simulink model "stm32f4_ds3231_configure_demo"  (Simulink 7.3)
settings: Solver=FixedStepDiscrete  SolverMode=SingleTasking  StartTime=0.0  StopTime=10.0  RelTol=1e-3
PreLoadFcn:
  | waijung.modelPreload; % Required for working with Waijung Blockset. Do not remove.
undefined symbols (not defined in the file): HSEOSC, Link, LQFP176, ST, STM32F417IG
libraries: simulink x94, amg_high_precision_rtc x5, stm32f4_io_lib x2, stm32f4_device_config_lib x1
(part 2 of 4)

== system stm32f4_ds3231_configure_demo/Display Date/Time/Display Hour ==
  In1 : Inport
  In2 : Inport  Port=2
  In3 : Inport  Port=3
  Data Type Conversion : DataTypeConversion  OutDataTypeMode=uint8  OutDataType=fixdt(1, 16)  OutScaling=2^0  OutDataTypeStr=uint8
  Logical Operator : Logic  Inputs=3  AllPortsSameDT=off  OutDataTypeMode=boolean  LogicDataType=fixdt(0, 8)  OutDataTypeStr=boolean
  Switch : Switch  Criteria=u2 ~= 0  OutDataType=fixdt(1, 16)  OutScaling=2^0
  Volatile Data Storage Read : S-Function  FunctionName=waijung_vdata_read  Parameters=storagename,varname,sampletime,sampletimestr,blockid,storagetype,storagetypestr  EnableBusSupport=off  mask(waijung_vdata_read){storagename=str_blank2, varname=CharacterLCDSetupVolatileDataStorage7_str_blank2, sampletime=inf, sampletimestr=0.01, blockid=DisplayDateTimeDisplayHourVolatileDataStorageRead, storagetype=string, storagetypestr=uint32_t}
      mask prompts: storagename "Storage Name"; varname "Variable name"; sampletime "Sample time (sec)"; sampletimestr "Compiled sample time (sec) in string"; storagetype "Data type"; storagetypestr "Data type string"
      mask help: This block implements read data from a buffer.
      mask init:
      | waijung_vdata_read_callback('init');
      mask Help: web(fullfile(waijungdocroot,'waijung_vdata_read.htm'))
      mask StyleString: popup(str_hour|str_month|str_year|str_minute|str_second|str_blank2|LCD_Buffer|str_date),edit,edit,edit,edit,edit,edit
      mask CallbackString: waijung_vdata_read_callback('storagename');|waijung_vdata_read_callback('varname');|waijung_vdata_read_callback('sampletime');|waijung_vdata_read_callback('sampletimestr');|waijung_vdata_read_callback('blockid');|waijung_vdata_read_callback('storagetype');|
      mask Display: text(0.05, 0.5, 'Buffer: str_blank2','ver','middle','hor','left');port_label('output',1,'D1(string)')
  Volatile Data Storage Read1 : S-Function  FunctionName=waijung_vdata_read  Parameters=storagename,varname,sampletime,sampletimestr,blockid,storagetype,storagetypestr  EnableBusSupport=off  mask(waijung_vdata_read){storagename=str_hour, varname=CharacterLCDSetupVolatileDataStorage1_str_hour, sampletime=inf, sampletimestr=0.01, blockid=DisplayDateTimeDisplayHourVolatileDataStorageRead1, storagetype=string, storagetypestr=uint32_t}
      mask prompts: storagename "Storage Name"; varname "Variable name"; sampletime "Sample time (sec)"; sampletimestr "Compiled sample time (sec) in string"; storagetype "Data type"; storagetypestr "Data type string"
      mask help: This block implements read data from a buffer.
      mask init:
      | waijung_vdata_read_callback('init');
      mask Help: web(fullfile(waijungdocroot,'waijung_vdata_read.htm'))
      mask StyleString: popup(str_hour|str_month|str_year|str_minute|str_second|str_blank2|LCD_Buffer|str_date),edit,edit,edit,edit,edit,edit
      mask CallbackString: waijung_vdata_read_callback('storagename');|waijung_vdata_read_callback('varname');|waijung_vdata_read_callback('sampletime');|waijung_vdata_read_callback('sampletimestr');|waijung_vdata_read_callback('blockid');|waijung_vdata_read_callback('storagetype');|
      mask Display: text(0.05, 0.5, 'Buffer: str_hour','ver','middle','hor','left');port_label('output',1,'D1(string)')
  Out1 : Outport
  wires:
  In3/1 -> Logical Operator/3
  Switch/1 -> Out1/1
  In2/1 -> Logical Operator/2
  In1/1 -> Logical Operator/1
  Volatile Data Storage Read1/1 -> Switch/3
  Volatile Data Storage Read/1 -> Switch/1
  Logical Operator/1 -> Data Type Conversion/1
  Data Type Conversion/1 -> Switch/2

== system stm32f4_ds3231_configure_demo/Display Date/Time/Display Minute ==
  In1 : Inport
  In2 : Inport  Port=2
  In3 : Inport  Port=3
  Data Type Conversion : DataTypeConversion  OutDataTypeMode=uint8  OutDataType=fixdt(1, 16)  OutScaling=2^0  OutDataTypeStr=uint8
  Logical Operator : Logic  Inputs=3  AllPortsSameDT=off  OutDataTypeMode=boolean  LogicDataType=fixdt(0, 8)  OutDataTypeStr=boolean
  Switch : Switch  Criteria=u2 ~= 0  OutDataType=fixdt(1, 16)  OutScaling=2^0
  Volatile Data Storage Read : S-Function  FunctionName=waijung_vdata_read  Parameters=storagename,varname,sampletime,sampletimestr,blockid,storagetype,storagetypestr  EnableBusSupport=off  mask(waijung_vdata_read){storagename=str_blank2, varname=CharacterLCDSetupVolatileDataStorage7_str_blank2, sampletime=inf, sampletimestr=0.01, blockid=DisplayDateTimeDisplayMinuteVolatileDataStorageRead, storagetype=string, storagetypestr=uint32_t}
      mask prompts: storagename "Storage Name"; varname "Variable name"; sampletime "Sample time (sec)"; sampletimestr "Compiled sample time (sec) in string"; storagetype "Data type"; storagetypestr "Data type string"
      mask help: This block implements read data from a buffer.
      mask init:
      | waijung_vdata_read_callback('init');
      mask Help: web(fullfile(waijungdocroot,'waijung_vdata_read.htm'))
      mask StyleString: popup(str_hour|str_month|str_year|str_minute|str_second|str_blank2|LCD_Buffer|str_date),edit,edit,edit,edit,edit,edit
      mask CallbackString: waijung_vdata_read_callback('storagename');|waijung_vdata_read_callback('varname');|waijung_vdata_read_callback('sampletime');|waijung_vdata_read_callback('sampletimestr');|waijung_vdata_read_callback('blockid');|waijung_vdata_read_callback('storagetype');|
      mask Display: text(0.05, 0.5, 'Buffer: str_blank2','ver','middle','hor','left');port_label('output',1,'D1(string)')
  Volatile Data Storage Read1 : S-Function  FunctionName=waijung_vdata_read  Parameters=storagename,varname,sampletime,sampletimestr,blockid,storagetype,storagetypestr  EnableBusSupport=off  mask(waijung_vdata_read){storagename=str_minute, varname=CharacterLCDSetupVolatileDataStorage4_str_minute, sampletime=inf, sampletimestr=0.01, blockid=DisplayDateTimeDisplayMinuteVolatileDataStorageRead1, storagetype=string, storagetypestr=uint32_t}
      mask prompts: storagename "Storage Name"; varname "Variable name"; sampletime "Sample time (sec)"; sampletimestr "Compiled sample time (sec) in string"; storagetype "Data type"; storagetypestr "Data type string"
      mask help: This block implements read data from a buffer.
      mask init:
      | waijung_vdata_read_callback('init');
      mask Help: web(fullfile(waijungdocroot,'waijung_vdata_read.htm'))
      mask StyleString: popup(str_hour|str_month|str_year|str_minute|str_second|str_blank2|LCD_Buffer|str_date),edit,edit,edit,edit,edit,edit
      mask CallbackString: waijung_vdata_read_callback('storagename');|waijung_vdata_read_callback('varname');|waijung_vdata_read_callback('sampletime');|waijung_vdata_read_callback('sampletimestr');|waijung_vdata_read_callback('blockid');|waijung_vdata_read_callback('storagetype');|
      mask Display: text(0.05, 0.5, 'Buffer: str_minute','ver','middle','hor','left');port_label('output',1,'D1(string)')
  Out1 : Outport
  wires:
  Data Type Conversion/1 -> Switch/2
  Logical Operator/1 -> Data Type Conversion/1
  Volatile Data Storage Read/1 -> Switch/1
  Volatile Data Storage Read1/1 -> Switch/3
  In1/1 -> Logical Operator/1
  In2/1 -> Logical Operator/2
  Switch/1 -> Out1/1
  In3/1 -> Logical Operator/3

== system stm32f4_ds3231_configure_demo/Display Date/Time/Display Month ==
  In1 : Inport
  In2 : Inport  Port=2
  In3 : Inport  Port=3
  Data Type Conversion : DataTypeConversion  OutDataTypeMode=uint8  OutDataType=fixdt(1, 16)  OutScaling=2^0  OutDataTypeStr=uint8
  Logical Operator : Logic  Inputs=3  AllPortsSameDT=off  OutDataTypeMode=boolean  LogicDataType=fixdt(0, 8)  OutDataTypeStr=boolean
  Switch : Switch  Criteria=u2 ~= 0  OutDataType=fixdt(1, 16)  OutScaling=2^0
  Volatile Data Storage Read : S-Function  FunctionName=waijung_vdata_read  Parameters=storagename,varname,sampletime,sampletimestr,blockid,storagetype,storagetypestr  EnableBusSupport=off  mask(waijung_vdata_read){storagename=str_blank2, varname=CharacterLCDSetupVolatileDataStorage7_str_blank2, sampletime=inf, sampletimestr=0.01, blockid=DisplayDateTimeDisplayMonthVolatileDataStorageRead, storagetype=string, storagetypestr=uint32_t}
      mask prompts: storagename "Storage Name"; varname "Variable name"; sampletime "Sample time (sec)"; sampletimestr "Compiled sample time (sec) in string"; storagetype "Data type"; storagetypestr "Data type string"
      mask help: This block implements read data from a buffer.
      mask init:
      | waijung_vdata_read_callback('init');
      mask Help: web(fullfile(waijungdocroot,'waijung_vdata_read.htm'))
      mask StyleString: popup(str_hour|str_month|str_year|str_minute|str_second|str_blank2|LCD_Buffer|str_date),edit,edit,edit,edit,edit,edit
      mask CallbackString: waijung_vdata_read_callback('storagename');|waijung_vdata_read_callback('varname');|waijung_vdata_read_callback('sampletime');|waijung_vdata_read_callback('sampletimestr');|waijung_vdata_read_callback('blockid');|waijung_vdata_read_callback('storagetype');|
      mask Display: text(0.05, 0.5, 'Buffer: str_blank2','ver','middle','hor','left');port_label('output',1,'D1(string)')
  Volatile Data Storage Read1 : S-Function  FunctionName=waijung_vdata_read  Parameters=storagename,varname,sampletime,sampletimestr,blockid,storagetype,storagetypestr  EnableBusSupport=off  mask(waijung_vdata_read){storagename=str_month, varname=CharacterLCDSetupVolatileDataStorage2_str_month, sampletime=inf, sampletimestr=0.01, blockid=DisplayDateTimeDisplayMonthVolatileDataStorageRead1, storagetype=string, storagetypestr=uint32_t}
      mask prompts: storagename "Storage Name"; varname "Variable name"; sampletime "Sample time (sec)"; sampletimestr "Compiled sample time (sec) in string"; storagetype "Data type"; storagetypestr "Data type string"
      mask help: This block implements read data from a buffer.
      mask init:
      | waijung_vdata_read_callback('init');
      mask Help: web(fullfile(waijungdocroot,'waijung_vdata_read.htm'))
      mask StyleString: popup(str_hour|str_month|str_year|str_minute|str_second|str_blank2|LCD_Buffer|str_date),edit,edit,edit,edit,edit,edit
      mask CallbackString: waijung_vdata_read_callback('storagename');|waijung_vdata_read_callback('varname');|waijung_vdata_read_callback('sampletime');|waijung_vdata_read_callback('sampletimestr');|waijung_vdata_read_callback('blockid');|waijung_vdata_read_callback('storagetype');|
      mask Display: text(0.05, 0.5, 'Buffer: str_month','ver','middle','hor','left');port_label('output',1,'D1(string)')
  Out1 : Outport
  wires:
  In3/1 -> Logical Operator/3
  Switch/1 -> Out1/1
  In2/1 -> Logical Operator/2
  In1/1 -> Logical Operator/1
  Volatile Data Storage Read1/1 -> Switch/3
  Volatile Data Storage Read/1 -> Switch/1
  Logical Operator/1 -> Data Type Conversion/1
  Data Type Conversion/1 -> Switch/2

== system stm32f4_ds3231_configure_demo/Display Date/Time/Display Second ==
  In1 : Inport
  In2 : Inport  Port=2
  In3 : Inport  Port=3
  Data Type Conversion : DataTypeConversion  OutDataTypeMode=uint8  OutDataType=fixdt(1, 16)  OutScaling=2^0  OutDataTypeStr=uint8
  Logical Operator : Logic  Inputs=3  AllPortsSameDT=off  OutDataTypeMode=boolean  LogicDataType=fixdt(0, 8)  OutDataTypeStr=boolean
  Switch : Switch  Criteria=u2 ~= 0  OutDataType=fixdt(1, 16)  OutScaling=2^0
  Volatile Data Storage Read : S-Function  FunctionName=waijung_vdata_read  Parameters=storagename,varname,sampletime,sampletimestr,blockid,storagetype,storagetypestr  EnableBusSupport=off  mask(waijung_vdata_read){storagename=str_blank2, varname=CharacterLCDSetupVolatileDataStorage7_str_blank2, sampletime=inf, sampletimestr=0.01, blockid=DisplayDateTimeDisplaySecondVolatileDataStorageRead, storagetype=string, storagetypestr=uint32_t}
      mask prompts: storagename "Storage Name"; varname "Variable name"; sampletime "Sample time (sec)"; sampletimestr "Compiled sample time (sec) in string"; storagetype "Data type"; storagetypestr "Data type string"
      mask help: This block implements read data from a buffer.
      mask init:
      | waijung_vdata_read_callback('init');
      mask Help: web(fullfile(waijungdocroot,'waijung_vdata_read.htm'))
      mask StyleString: popup(str_hour|str_month|str_year|str_minute|str_second|str_blank2|LCD_Buffer|str_date),edit,edit,edit,edit,edit,edit
      mask CallbackString: waijung_vdata_read_callback('storagename');|waijung_vdata_read_callback('varname');|waijung_vdata_read_callback('sampletime');|waijung_vdata_read_callback('sampletimestr');|waijung_vdata_read_callback('blockid');|waijung_vdata_read_callback('storagetype');|
      mask Display: text(0.05, 0.5, 'Buffer: str_blank2','ver','middle','hor','left');port_label('output',1,'D1(string)')
  Volatile Data Storage Read1 : S-Function  FunctionName=waijung_vdata_read  Parameters=storagename,varname,sampletime,sampletimestr,blockid,storagetype,storagetypestr  EnableBusSupport=off  mask(waijung_vdata_read){storagename=str_second, varname=CharacterLCDSetupVolatileDataStorage5_str_second, sampletime=inf, sampletimestr=0.01, blockid=DisplayDateTimeDisplaySecondVolatileDataStorageRead1, storagetype=string, storagetypestr=uint32_t}
      mask prompts: storagename "Storage Name"; varname "Variable name"; sampletime "Sample time (sec)"; sampletimestr "Compiled sample time (sec) in string"; storagetype "Data type"; storagetypestr "Data type string"
      mask help: This block implements read data from a buffer.
      mask init:
      | waijung_vdata_read_callback('init');
      mask Help: web(fullfile(waijungdocroot,'waijung_vdata_read.htm'))
      mask StyleString: popup(str_hour|str_month|str_year|str_minute|str_second|str_blank2|LCD_Buffer|str_date),edit,edit,edit,edit,edit,edit
      mask CallbackString: waijung_vdata_read_callback('storagename');|waijung_vdata_read_callback('varname');|waijung_vdata_read_callback('sampletime');|waijung_vdata_read_callback('sampletimestr');|waijung_vdata_read_callback('blockid');|waijung_vdata_read_callback('storagetype');|
      mask Display: text(0.05, 0.5, 'Buffer: str_second','ver','middle','hor','left');port_label('output',1,'D1(string)')
  Out1 : Outport
  wires:
  In3/1 -> Logical Operator/3
  Switch/1 -> Out1/1
  In2/1 -> Logical Operator/2
  In1/1 -> Logical Operator/1
  Volatile Data Storage Read1/1 -> Switch/3
  Volatile Data Storage Read/1 -> Switch/1
  Logical Operator/1 -> Data Type Conversion/1
  Data Type Conversion/1 -> Switch/2

== system stm32f4_ds3231_configure_demo/Display Date/Time/Display Year ==
  In1 : Inport
  In2 : Inport  Port=2
  In3 : Inport  Port=3
  Data Type Conversion : DataTypeConversion  OutDataTypeMode=uint8  OutDataType=fixdt(1, 16)  OutScaling=2^0  OutDataTypeStr=uint8
  Logical Operator : Logic  Inputs=3  AllPortsSameDT=off  OutDataTypeMode=boolean  LogicDataType=fixdt(0, 8)  OutDataTypeStr=boolean
  Switch : Switch  Criteria=u2 ~= 0  OutDataType=fixdt(1, 16)  OutScaling=2^0
  Volatile Data Storage Read : S-Function  FunctionName=waijung_vdata_read  Parameters=storagename,varname,sampletime,sampletimestr,blockid,storagetype,storagetypestr  EnableBusSupport=off  mask(waijung_vdata_read){storagename=str_blank2, varname=CharacterLCDSetupVolatileDataStorage7_str_blank2, sampletime=inf, sampletimestr=0.01, blockid=DisplayDateTimeDisplayYearVolatileDataStorageRead, storagetype=string, storagetypestr=uint32_t}
      mask prompts: storagename "Storage Name"; varname "Variable name"; sampletime "Sample time (sec)"; sampletimestr "Compiled sample time (sec) in string"; storagetype "Data type"; storagetypestr "Data type string"
      mask help: This block implements read data from a buffer.
      mask init:
      | waijung_vdata_read_callback('init');
      mask Help: web(fullfile(waijungdocroot,'waijung_vdata_read.htm'))
      mask StyleString: popup(str_hour|str_month|str_year|str_minute|str_second|str_blank2|LCD_Buffer|str_date),edit,edit,edit,edit,edit,edit
      mask CallbackString: waijung_vdata_read_callback('storagename');|waijung_vdata_read_callback('varname');|waijung_vdata_read_callback('sampletime');|waijung_vdata_read_callback('sampletimestr');|waijung_vdata_read_callback('blockid');|waijung_vdata_read_callback('storagetype');|
      mask Display: text(0.05, 0.5, 'Buffer: str_blank2','ver','middle','hor','left');port_label('output',1,'D1(string)')
  Volatile Data Storage Read1 : S-Function  FunctionName=waijung_vdata_read  Parameters=storagename,varname,sampletime,sampletimestr,blockid,storagetype,storagetypestr  EnableBusSupport=off  mask(waijung_vdata_read){storagename=str_year, varname=CharacterLCDSetupVolatileDataStorage3_str_year, sampletime=inf, sampletimestr=0.01, blockid=DisplayDateTimeDisplayYearVolatileDataStorageRead1, storagetype=string, storagetypestr=uint32_t}
      mask prompts: storagename "Storage Name"; varname "Variable name"; sampletime "Sample time (sec)"; sampletimestr "Compiled sample time (sec) in string"; storagetype "Data type"; storagetypestr "Data type string"
      mask help: This block implements read data from a buffer.
      mask init:
      | waijung_vdata_read_callback('init');
      mask Help: web(fullfile(waijungdocroot,'waijung_vdata_read.htm'))
      mask StyleString: popup(str_hour|str_month|str_year|str_minute|str_second|str_blank2|LCD_Buffer|str_date),edit,edit,edit,edit,edit,edit
      mask CallbackString: waijung_vdata_read_callback('storagename');|waijung_vdata_read_callback('varname');|waijung_vdata_read_callback('sampletime');|waijung_vdata_read_callback('sampletimestr');|waijung_vdata_read_callback('blockid');|waijung_vdata_read_callback('storagetype');|
      mask Display: text(0.05, 0.5, 'Buffer: str_year','ver','middle','hor','left');port_label('output',1,'D1(string)')
  Out1 : Outport
  wires:
  Data Type Conversion/1 -> Switch/2
  Logical Operator/1 -> Data Type Conversion/1
  Volatile Data Storage Read/1 -> Switch/1
  Volatile Data Storage Read1/1 -> Switch/3
  In1/1 -> Logical Operator/1
  In2/1 -> Logical Operator/2
  Switch/1 -> Out1/1
  In3/1 -> Logical Operator/3

== system stm32f4_ds3231_configure_demo/Display Date/Time/Get Date as String ==
  In1 : Inport
  DS3231 Get Date : Subsystem  mask{blockfunction=date, module=1}
      mask prompts: blockfunction "Function"; module "I2C module"
      mask init:
      | amg_high_precision_rtc_callback('init');
      mask StyleString: popup(temp|time|date),popup(1|2|3)
      mask CallbackString: |amg_high_precision_rtc_callback('module');
      mask Display: text(0.5, 0.5, 'Port: I2C1','ver','middle','hor','center');port_label('input', 1,'SlvAddr');port_label('output', 1,'Status');port_label('output', 2,'Day(1-7)');port_label('output', 3,'Date(1-31)');port_label('output', 4,'Month(1-12)');port_label('output', 5,'Year(0-99)');
  Printf1 : S-Function  FunctionName=waijung_printf  Parameters=storagename,printfformat,formatcode,varname,sampletime,sampletimestr,blockid  EnableBusSupport=off  mask(waijung_printf){storagename=str_date, printfformat=%2u/, formatcode=u, varname=CharacterLCDSetupVolatileDataStorage9_str_date, sampletime=-1, sampletimestr=0.01, blockid=DisplayDateTimeGetDateasStringPrintf1}
      mask prompts: storagename "Storage Name"; printfformat "Printf format"; formatcode "Printf format code"; varname "Variable name"; sampletime "Sample time (sec)"; sampletimestr "Compiled sample time (sec) in string"
      mask help: This block implements printf command.
      mask init:
      | waijung_printf_callback('init');
      mask Help: web(fullfile(waijungdocroot,'waijung_printf.htm'))
      mask StyleString: popup(str_hour|str_month|str_year|str_minute|str_second|str_blank2|LCD_Buffer|str_date),edit,edit,edit,edit,edit,edit
      mask CallbackString: waijung_printf_callback('storagename');|waijung_printf_callback('printfformat');|waijung_printf_callback('formatcode');|waijung_printf_callback('varname');|waijung_printf_callback('sampletime');|waijung_printf_callback('sampletimestr');|waijung_printf_callback('blockid');
      mask Display: text(0.95, 0.5, 'Buffer: str_date\nTs (sec): 0.01','ver','middle','hor','right');port_label('input',1,'D1(%u)');
  Printf2 : S-Function  FunctionName=waijung_printf  Parameters=storagename,printfformat,formatcode,varname,sampletime,sampletimestr,blockid  EnableBusSupport=off  mask(waijung_printf){storagename=str_month, printfformat=%2u/, formatcode=u, varname=CharacterLCDSetupVolatileDataStorage2_str_month, sampletime=-1, sampletimestr=0.01, blockid=DisplayDateTimeGetDateasStringPrintf2}
      mask prompts: storagename "Storage Name"; printfformat "Printf format"; formatcode "Printf format code"; varname "Variable name"; sampletime "Sample time (sec)"; sampletimestr "Compiled sample time (sec) in string"
      mask help: This block implements printf command.
      mask init:
      | waijung_printf_callback('init');
      mask Help: web(fullfile(waijungdocroot,'waijung_printf.htm'))
      mask StyleString: popup(str_hour|str_month|str_year|str_minute|str_second|str_blank2|LCD_Buffer|str_date),edit,edit,edit,edit,edit,edit
      mask CallbackString: waijung_printf_callback('storagename');|waijung_printf_callback('printfformat');|waijung_printf_callback('formatcode');|waijung_printf_callback('varname');|waijung_printf_callback('sampletime');|waijung_printf_callback('sampletimestr');|waijung_printf_callback('blockid');
      mask Display: text(0.95, 0.5, 'Buffer: str_month\nTs (sec): 0.01','ver','middle','hor','right');port_label('input',1,'D1(%u)');
  Printf3 : S-Function  FunctionName=waijung_printf  Parameters=storagename,printfformat,formatcode,varname,sampletime,sampletimestr,blockid  EnableBusSupport=off  mask(waijung_printf){storagename=str_year, printfformat=%2u, formatcode=u, varname=CharacterLCDSetupVolatileDataStorage3_str_year, sampletime=-1, sampletimestr=0.01, blockid=DisplayDateTimeGetDateasStringPrintf3}
      mask prompts: storagename "Storage Name"; printfformat "Printf format"; formatcode "Printf format code"; varname "Variable name"; sampletime "Sample time (sec)"; sampletimestr "Compiled sample time (sec) in string"
      mask help: This block implements printf command.
      mask init:
      | waijung_printf_callback('init');
      mask Help: web(fullfile(waijungdocroot,'waijung_printf.htm'))
      mask StyleString: popup(str_hour|str_month|str_year|str_minute|str_second|str_blank2|LCD_Buffer|str_date),edit,edit,edit,edit,edit,edit
      mask CallbackString: waijung_printf_callback('storagename');|waijung_printf_callback('printfformat');|waijung_printf_callback('formatcode');|waijung_printf_callback('varname');|waijung_printf_callback('sampletime');|waijung_printf_callback('sampletimestr');|waijung_printf_callback('blockid');
      mask Display: text(0.95, 0.5, 'Buffer: str_year\nTs (sec): 0.01','ver','middle','hor','right');port_label('input',1,'D1(%u)');
  Terminator : Terminator
  Terminator1 : Terminator
  wires:
  DS3231 Get Date/3(Date) -> Printf1/1
  DS3231 Get Date/5(Year) -> Printf3/1
  DS3231 Get Date/4(Month) -> Printf2/1
  DS3231 Get Date/1(Status) -> Terminator/1
  DS3231 Get Date/2(Day) -> Terminator1/1
  In1/1 -> DS3231 Get Date/1(Slave Address)

== system stm32f4_ds3231_configure_demo/Display Date/Time/Get Time as String ==
  In1 : Inport
  DS3231 Get Time : Subsystem  mask{blockfunction=time, module=1}
      mask prompts: blockfunction "Function"; module "I2C module"
      mask init:
      | amg_high_precision_rtc_callback('init');
      mask StyleString: popup(temp|time|date),popup(1|2|3)
      mask CallbackString: |amg_high_precision_rtc_callback('module');
      mask Display: text(0.5, 0.5, 'Port: I2C1','ver','middle','hor','center');port_label('input', 1,'SlvAddr');port_label('output', 1,'Status');port_label('output', 2,'Hour(0-11/23)');port_label('output', 3,'Minute(0-59)');port_label('output', 4,'Second(0-59)');port_label('output', 5,'AM(0)/PM(1)');
  Printf4 : S-Function  FunctionName=waijung_printf  Parameters=storagename,printfformat,formatcode,varname,sampletime,sampletimestr,blockid  EnableBusSupport=off  mask(waijung_printf){storagename=str_hour, printfformat=%2u:, formatcode=u, varname=CharacterLCDSetupVolatileDataStorage1_str_hour, sampletime=-1, sampletimestr=0.01, blockid=DisplayDateTimeGetTimeasStringPrintf4}
      mask prompts: storagename "Storage Name"; printfformat "Printf format"; formatcode "Printf format code"; varname "Variable name"; sampletime "Sample time (sec)"; sampletimestr "Compiled sample time (sec) in string"
      mask help: This block implements printf command.
      mask init:
      | waijung_printf_callback('init');
      mask Help: web(fullfile(waijungdocroot,'waijung_printf.htm'))
      mask StyleString: popup(str_hour|str_month|str_year|str_minute|str_second|str_blank2|LCD_Buffer|str_date),edit,edit,edit,edit,edit,edit
      mask CallbackString: waijung_printf_callback('storagename');|waijung_printf_callback('printfformat');|waijung_printf_callback('formatcode');|waijung_printf_callback('varname');|waijung_printf_callback('sampletime');|waijung_printf_callback('sampletimestr');|waijung_printf_callback('blockid');
      mask Display: text(0.95, 0.5, 'Buffer: str_hour\nTs (sec): 0.01','ver','middle','hor','right');port_label('input',1,'D1(%u)');
  Printf5 : S-Function  FunctionName=waijung_printf  Parameters=storagename,printfformat,formatcode,varname,sampletime,sampletimestr,blockid  EnableBusSupport=off  mask(waijung_printf){storagename=str_minute, printfformat=%2u:, formatcode=u, varname=CharacterLCDSetupVolatileDataStorage4_str_minute, sampletime=-1, sampletimestr=0.01, blockid=DisplayDateTimeGetTimeasStringPrintf5}
      mask prompts: storagename "Storage Name"; printfformat "Printf format"; formatcode "Printf format code"; varname "Variable name"; sampletime "Sample time (sec)"; sampletimestr "Compiled sample time (sec) in string"
      mask help: This block implements printf command.
      mask init:
      | waijung_printf_callback('init');
      mask Help: web(fullfile(waijungdocroot,'waijung_printf.htm'))
      mask StyleString: popup(str_hour|str_month|str_year|str_minute|str_second|str_blank2|LCD_Buffer|str_date),edit,edit,edit,edit,edit,edit
      mask CallbackString: waijung_printf_callback('storagename');|waijung_printf_callback('printfformat');|waijung_printf_callback('formatcode');|waijung_printf_callback('varname');|waijung_printf_callback('sampletime');|waijung_printf_callback('sampletimestr');|waijung_printf_callback('blockid');
      mask Display: text(0.95, 0.5, 'Buffer: str_minute\nTs (sec): 0.01','ver','middle','hor','right');port_label('input',1,'D1(%u)');
  Printf6 : S-Function  FunctionName=waijung_printf  Parameters=storagename,printfformat,formatcode,varname,sampletime,sampletimestr,blockid  EnableBusSupport=off  mask(waijung_printf){storagename=str_second, printfformat=%2u, formatcode=u, varname=CharacterLCDSetupVolatileDataStorage5_str_second, sampletime=-1, sampletimestr=0.01, blockid=DisplayDateTimeGetTimeasStringPrintf6}
      mask prompts: storagename "Storage Name"; printfformat "Printf format"; formatcode "Printf format code"; varname "Variable name"; sampletime "Sample time (sec)"; sampletimestr "Compiled sample time (sec) in string"
      mask help: This block implements printf command.
      mask init:
      | waijung_printf_callback('init');
      mask Help: web(fullfile(waijungdocroot,'waijung_printf.htm'))
      mask StyleString: popup(str_hour|str_month|str_year|str_minute|str_second|str_blank2|LCD_Buffer|str_date),edit,edit,edit,edit,edit,edit
      mask CallbackString: waijung_printf_callback('storagename');|waijung_printf_callback('printfformat');|waijung_printf_callback('formatcode');|waijung_printf_callback('varname');|waijung_printf_callback('sampletime');|waijung_printf_callback('sampletimestr');|waijung_printf_callback('blockid');
      mask Display: text(0.95, 0.5, 'Buffer: str_second\nTs (sec): 0.01','ver','middle','hor','right');port_label('input',1,'D1(%u)');
  Terminator2 : Terminator
  Terminator3 : Terminator
  wires:
  DS3231 Get Time/4(Second) -> Printf6/1
  DS3231 Get Time/3(Minute) -> Printf5/1
  DS3231 Get Time/2(Hour) -> Printf4/1
  DS3231 Get Time/1(Status) -> Terminator2/1
  DS3231 Get Time/5(AM/PM) -> Terminator3/1
  In1/1 -> DS3231 Get Time/1(Slave Address)

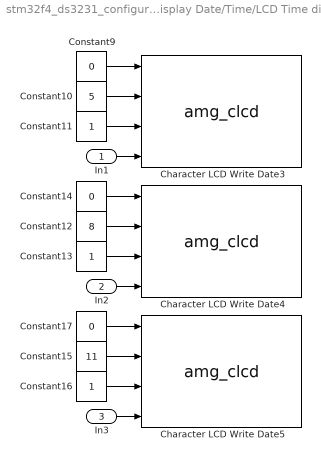
== system stm32f4_ds3231_configure_demo/Display Date/Time/LCD Time display ==
  In1 : Inport
  In2 : Inport  Port=2
  In3 : Inport  Port=3
  Character LCD Write Date3 : S-Function  FunctionName=amg_clcd  Parameters=module,configuration,inputtypearray,outputtypearray,confstr,sampletime,sampletimestr,blockid  EnableBusSupport=off  mask(amg_clcd){configuration=Transaction, module=1, model=amg CLCD Std, interface=4-bits, linecount=4, columncount=20, gpiotype=Push-pull, controlport=E, control_rs=15, control_rw=13, control_en=11, dataport=A, data0=7, data1=5, data2=3, data3=1, usestringbuffer=off, stringbuffer=<empty>, varname=, inputtypearray=[4 -1 -1 -1 -1], outputtypearray=[0], confstr=["4","4","20","PP","E","15","11","13","","A","","","","","7","5","3","1","0","","1","0","0","0","1","0","0","0","0","stm32f4"], sampletime=-1, sampletimestr=0.01, blockid=DisplayDateTimeLCDTimedisplayCharacterLCDWriteDate3}
      mask prompts: model "LCD model:"; linecount "Number of lines:"; columncount "Number of columns:"; gpiotype "GPIO Output type:"; controlport "GPIO control port:"; control_rs "GPIO control pin, RS:"; control_rw "GPIO control pin, RW:"; control_en "GPIO control pin, EN:"; dataport "GPIO data D[7:4] port"; data0 "GPIO data pin, D4:"; data1 "GPIO data pin, D5:"; data2 "GPIO data pin, D6:"; data3 "GPIO data pin, D7:"; usestringbuffer "Use string buffer"; stringbuffer "String buffer"; varname "Variable name"; inputtypearray "Input type array"; outputtypearray "Output type array"; confstr "Configuration string"; sampletime "Sample time (sec)"; sampletimestr "Compiled sample time (sec) in string"
      mask help:
      | Note for cmd:
      | 1 - Clear LCD Line before write.
      | 0 or otherwise - Write into LCD Line with existing data.
      mask init:
      | amg_clcd_callback('init');
      mask Help: web(fullfile(waijungdocroot,'amg_clcd_write.htm'), '-browser')
      mask StyleString: popup(Setup|Transaction),popup(1|2|3|4),popup(amg CLCD Std),popup(4-bits),edit,edit,popup(Push-pull|Open-drain),popup(A|B|C|D|E|F|G|H|I),popup(0|1|2|3|4|5|6|7|8|9|10|11|12|13|14|15),popup(0|1|2|3|4|5|6|7|8|9|10|11|12|13|14|15),popup(0|1|2|3|4|5|6|7|8|9|10|11|12|13|14|15),popup(A|B|C|D|E|F|G|H|I),popup(0|1|2|3|4|5|6|7|8|9|10|11|12|13|14|15),popup(0|1|2|3|4|5|6|7|8|9|10|11|12|13|14|15),popup(0|1|2|3|4|5|6|7|8|9|10|11|12|13|14|15),popup(0|1|2|3|4|5|6|7|8|9|10|11|12|13|14|15),checkbox,popup(str_hour|str_month|str_year|str_minute|str_second|str_blank2|LCD_Buffer|str_date|<empty>),edit,edit,edit,edit,edit,edit,edit
      mask CallbackString: amg_clcd_callback('configuration');||||||||||||||||amg_clcd_callback('usestringbuffer');||amg_clcd_callback('varname');|||amg_clcd_callback('confstr');|amg_clcd_callback('sampletime');|amg_clcd_callback('sampletimestr');|amg_clcd_callback('blockid');
      mask Display: text(0.5, 0.5, 'Module: CLCD1 (Write)\nTs (sec): 0.01','ver','middle','hor','center');port_label('input', 1,'cmd');port_label('input', 2,'xpos');port_label('input', 3,'ypos');port_label('input', 4,'str');
  Character LCD Write Date4 : S-Function  FunctionName=amg_clcd  Parameters=module,configuration,inputtypearray,outputtypearray,confstr,sampletime,sampletimestr,blockid  EnableBusSupport=off  mask(amg_clcd){configuration=Transaction, module=1, model=amg CLCD Std, interface=4-bits, linecount=4, columncount=20, gpiotype=Push-pull, controlport=E, control_rs=15, control_rw=13, control_en=11, dataport=A, data0=7, data1=5, data2=3, data3=1, usestringbuffer=off, stringbuffer=<empty>, varname=, inputtypearray=[4 -1 -1 -1 -1], outputtypearray=[0], confstr=["4","4","20","PP","E","15","11","13","","A","","","","","7","5","3","1","0","","1","0","0","0","1","0","0","0","0","stm32f4"], sampletime=-1, sampletimestr=0.01, blockid=DisplayDateTimeLCDTimedisplayCharacterLCDWriteDate4}
      mask prompts: model "LCD model:"; linecount "Number of lines:"; columncount "Number of columns:"; gpiotype "GPIO Output type:"; controlport "GPIO control port:"; control_rs "GPIO control pin, RS:"; control_rw "GPIO control pin, RW:"; control_en "GPIO control pin, EN:"; dataport "GPIO data D[7:4] port"; data0 "GPIO data pin, D4:"; data1 "GPIO data pin, D5:"; data2 "GPIO data pin, D6:"; data3 "GPIO data pin, D7:"; usestringbuffer "Use string buffer"; stringbuffer "String buffer"; varname "Variable name"; inputtypearray "Input type array"; outputtypearray "Output type array"; confstr "Configuration string"; sampletime "Sample time (sec)"; sampletimestr "Compiled sample time (sec) in string"
      mask help:
      | Note for cmd:
      | 1 - Clear LCD Line before write.
      | 0 or otherwise - Write into LCD Line with existing data.
      mask init:
      | amg_clcd_callback('init');
      mask Help: web(fullfile(waijungdocroot,'amg_clcd_write.htm'), '-browser')
      mask StyleString: popup(Setup|Transaction),popup(1|2|3|4),popup(amg CLCD Std),popup(4-bits),edit,edit,popup(Push-pull|Open-drain),popup(A|B|C|D|E|F|G|H|I),popup(0|1|2|3|4|5|6|7|8|9|10|11|12|13|14|15),popup(0|1|2|3|4|5|6|7|8|9|10|11|12|13|14|15),popup(0|1|2|3|4|5|6|7|8|9|10|11|12|13|14|15),popup(A|B|C|D|E|F|G|H|I),popup(0|1|2|3|4|5|6|7|8|9|10|11|12|13|14|15),popup(0|1|2|3|4|5|6|7|8|9|10|11|12|13|14|15),popup(0|1|2|3|4|5|6|7|8|9|10|11|12|13|14|15),popup(0|1|2|3|4|5|6|7|8|9|10|11|12|13|14|15),checkbox,popup(str_hour|str_month|str_year|str_minute|str_second|str_blank2|LCD_Buffer|str_date|<empty>),edit,edit,edit,edit,edit,edit,edit
      mask CallbackString: amg_clcd_callback('configuration');||||||||||||||||amg_clcd_callback('usestringbuffer');||amg_clcd_callback('varname');|||amg_clcd_callback('confstr');|amg_clcd_callback('sampletime');|amg_clcd_callback('sampletimestr');|amg_clcd_callback('blockid');
      mask Display: text(0.5, 0.5, 'Module: CLCD1 (Write)\nTs (sec): 0.01','ver','middle','hor','center');port_label('input', 1,'cmd');port_label('input', 2,'xpos');port_label('input', 3,'ypos');port_label('input', 4,'str');
  Character LCD Write Date5 : S-Function  FunctionName=amg_clcd  Parameters=module,configuration,inputtypearray,outputtypearray,confstr,sampletime,sampletimestr,blockid  EnableBusSupport=off  mask(amg_clcd){configuration=Transaction, module=1, model=amg CLCD Std, interface=4-bits, linecount=4, columncount=20, gpiotype=Push-pull, controlport=E, control_rs=15, control_rw=13, control_en=11, dataport=A, data0=7, data1=5, data2=3, data3=1, usestringbuffer=off, stringbuffer=<empty>, varname=, inputtypearray=[4 -1 -1 -1 -1], outputtypearray=[0], confstr=["4","4","20","PP","E","15","11","13","","A","","","","","7","5","3","1","0","","1","0","0","0","1","0","0","0","0","stm32f4"], sampletime=-1, sampletimestr=0.01, blockid=DisplayDateTimeLCDTimedisplayCharacterLCDWriteDate5}
      mask prompts: model "LCD model:"; linecount "Number of lines:"; columncount "Number of columns:"; gpiotype "GPIO Output type:"; controlport "GPIO control port:"; control_rs "GPIO control pin, RS:"; control_rw "GPIO control pin, RW:"; control_en "GPIO control pin, EN:"; dataport "GPIO data D[7:4] port"; data0 "GPIO data pin, D4:"; data1 "GPIO data pin, D5:"; data2 "GPIO data pin, D6:"; data3 "GPIO data pin, D7:"; usestringbuffer "Use string buffer"; stringbuffer "String buffer"; varname "Variable name"; inputtypearray "Input type array"; outputtypearray "Output type array"; confstr "Configuration string"; sampletime "Sample time (sec)"; sampletimestr "Compiled sample time (sec) in string"
      mask help:
      | Note for cmd:
      | 1 - Clear LCD Line before write.
      | 0 or otherwise - Write into LCD Line with existing data.
      mask init:
      | amg_clcd_callback('init');
      mask Help: web(fullfile(waijungdocroot,'amg_clcd_write.htm'), '-browser')
      mask StyleString: popup(Setup|Transaction),popup(1|2|3|4),popup(amg CLCD Std),popup(4-bits),edit,edit,popup(Push-pull|Open-drain),popup(A|B|C|D|E|F|G|H|I),popup(0|1|2|3|4|5|6|7|8|9|10|11|12|13|14|15),popup(0|1|2|3|4|5|6|7|8|9|10|11|12|13|14|15),popup(0|1|2|3|4|5|6|7|8|9|10|11|12|13|14|15),popup(A|B|C|D|E|F|G|H|I),popup(0|1|2|3|4|5|6|7|8|9|10|11|12|13|14|15),popup(0|1|2|3|4|5|6|7|8|9|10|11|12|13|14|15),popup(0|1|2|3|4|5|6|7|8|9|10|11|12|13|14|15),popup(0|1|2|3|4|5|6|7|8|9|10|11|12|13|14|15),checkbox,popup(str_hour|str_month|str_year|str_minute|str_second|str_blank2|LCD_Buffer|str_date|<empty>),edit,edit,edit,edit,edit,edit,edit
      mask CallbackString: amg_clcd_callback('configuration');||||||||||||||||amg_clcd_callback('usestringbuffer');||amg_clcd_callback('varname');|||amg_clcd_callback('confstr');|amg_clcd_callback('sampletime');|amg_clcd_callback('sampletimestr');|amg_clcd_callback('blockid');
      mask Display: text(0.5, 0.5, 'Module: CLCD1 (Write)\nTs (sec): 0.01','ver','middle','hor','center');port_label('input', 1,'cmd');port_label('input', 2,'xpos');port_label('input', 3,'ypos');port_label('input', 4,'str');
  Constant10 : Constant  Value=5  OutDataTypeMode=uint8  OutDataType=fixdt(1, 16)  OutScaling=2^0  OutDataTypeStr=uint8
  Constant11 : Constant  OutDataTypeMode=uint8  OutDataType=fixdt(1, 16)  OutScaling=2^0  OutDataTypeStr=uint8
  Constant12 : Constant  Value=8  OutDataTypeMode=uint8  OutDataType=fixdt(1, 16)  OutScaling=2^0  OutDataTypeStr=uint8
  Constant13 : Constant  OutDataTypeMode=uint8  OutDataType=fixdt(1, 16)  OutScaling=2^0  OutDataTypeStr=uint8
  Constant14 : Constant  Value=0  OutDataTypeMode=uint8  OutDataType=fixdt(1, 16)  OutScaling=2^0  OutDataTypeStr=uint8
  Constant15 : Constant  Value=11  OutDataTypeMode=uint8  OutDataType=fixdt(1, 16)  OutScaling=2^0  OutDataTypeStr=uint8
  Constant16 : Constant  OutDataTypeMode=uint8  OutDataType=fixdt(1, 16)  OutScaling=2^0  OutDataTypeStr=uint8
  Constant17 : Constant  Value=0  OutDataTypeMode=uint8  OutDataType=fixdt(1, 16)  OutScaling=2^0  OutDataTypeStr=uint8
  Constant9 : Constant  Value=0  OutDataTypeMode=uint8  OutDataType=fixdt(1, 16)  OutScaling=2^0  OutDataTypeStr=uint8
  wires:
  Constant10/1 -> Character LCD Write Date3/2
  Constant11/1 -> Character LCD Write Date3/3
  Constant9/1 -> Character LCD Write Date3/1
  Constant12/1 -> Character LCD Write Date4/2
  Constant13/1 -> Character LCD Write Date4/3
  Constant14/1 -> Character LCD Write Date4/1
  Constant15/1 -> Character LCD Write Date5/2
  Constant16/1 -> Character LCD Write Date5/3
  Constant17/1 -> Character LCD Write Date5/1
  In1/1 -> Character LCD Write Date3/4
  In2/1 -> Character LCD Write Date4/4
  In3/1 -> Character LCD Write Date5/4
